simulink model "LTRTenzo"  (R2015a)
settings: Solver=ode23  StartTime=0.0  StopTime=10  RelTol=1e-3
values from neighbouring files (symbols this model uses):
  A0 = tenzo_min_nominale.a    [HTenzoV10.m]    (also in HTenzoV11.m; HTenzoV12.m; HTenzoV13.m; HTenzoV14.m)
  amplitudeNoise = 2    [HTenzoV10.m]    (also in HTenzoV11.m; HTenzoV12.m; HTenzoV13.m; HTenzoV14.m)
  amplitudePertIN = 0    [HTenzoV10.m]    (also in HTenzoV11.m; HTenzoV12.m; HTenzoV13.m; HTenzoV14.m)
  amplitudePertOut = 0    [HTenzoV10.m]    (also in HTenzoV11.m; HTenzoV12.m; HTenzoV13.m; HTenzoV14.m)
  B0 = tenzo_min_nominale.b    [HTenzoV10.m]    (also in HTenzoV11.m; HTenzoV12.m; HTenzoV13.m; HTenzoV14.m)
  C0 = tenzo_min_nominale.c    [HTenzoV10.m]    (also in HTenzoV11.m; HTenzoV12.m; HTenzoV13.m; HTenzoV14.m)
  cstPertIn = 0    [HTenzoV10.m]    (also in HTenzoV11.m; HTenzoV12.m; HTenzoV13.m; HTenzoV14.m)
  cstPertOut = 0    [HTenzoV10.m]    (also in HTenzoV11.m; HTenzoV12.m; HTenzoV13.m; HTenzoV14.m)
  D0 = tenzo_min_nominale.d    [HTenzoV10.m]    (also in HTenzoV11.m; HTenzoV12.m; HTenzoV13.m; HTenzoV14.m)
  KAoss = tenzo_min_nominale.a-L_3*tenzo_min_nominale.c    [HTenzoV12.m]    (also in HTenzoV13.m; HTenzoV14.m; HTenzoV20.m; HTenzoV21.m)
  KBossw = [tenzo_min_nominale.b-L_3*D L_3]    [HTenzoV12.m]    (also in HTenzoV13.m; HTenzoV14.m; HTenzoV20.m; HTenzoV21.m)
  KCoss = eye(size(Aoss,1))    [HTenzoV12.m]    (also in HTenzoV13.m; HTenzoV14.m; HTenzoV20.m; HTenzoV21.m)
  KDoss = zeros(size(Aoss,1),poss)    [HTenzoV12.m]    (also in HTenzoV13.m; HTenzoV14.m; HTenzoV20.m; HTenzoV21.m)
  Kopt = Kopt_3    [HTenzoV10.m]    (also in HTenzoV11.m; HTenzoV12.m; HTenzoV13.m; HTenzoV14.m)
  omegaNoise = 370    [HTenzoV10.m]    (also in HTenzoV11.m; HTenzoV12.m; HTenzoV13.m; HTenzoV14.m)
  omegaPertIN = 6    [HTenzoV10.m]    (also in HTenzoV11.m; HTenzoV12.m; HTenzoV13.m; HTenzoV14.m)
  omegaPertOut = 0.1    [HTenzoV10.m]    (also in HTenzoV11.m; HTenzoV12.m; HTenzoV13.m; HTenzoV14.m)
  randomAmpNoise = 1    [HTenzoV10.m]    (also in HTenzoV11.m; HTenzoV12.m; HTenzoV13.m; HTenzoV14.m)
undefined symbols (not defined in the file or in its folder): sigbuilder_block
settings Model: SimulationMode=accelerator  Creator=danilo  LastModifiedBy=userk
settings OptimizationCC: ExpressionDepthLimit=2147483647
settings DebuggingCC: UnderspecifiedInitializationDetection=Classic  MergeDetectMultiDrivingBlocksExec=none  SolverPrmCheckMsg=warning  FcnCallInpInsideContextMsg=UseLocalSettings  StateNameClashWarn=warning
settings GRTTargetCC: CombineOutputUpdateFcns=off  GRTInterface=on

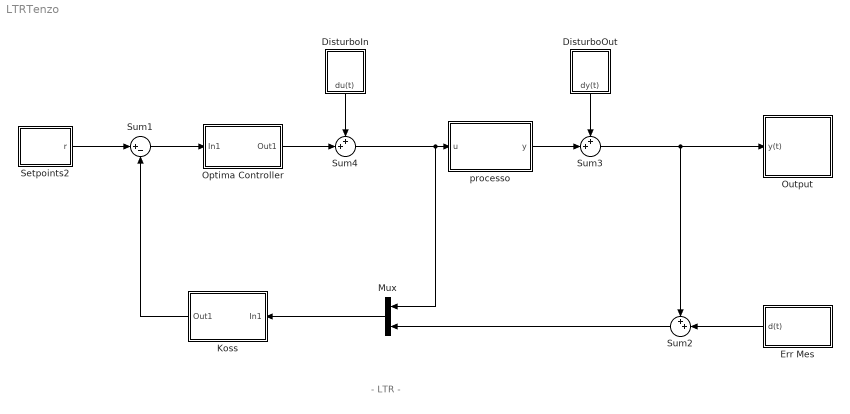
== system LTRTenzo ==
  note: - LTR -
  DisturboIn : Subsystem
  DisturboOut : Subsystem
  Err Mes : Subsystem
  Koss : Subsystem
  Mux : Mux  Inputs=2
  Optima Controller : Subsystem
  Output : Subsystem
  Setpoints2 : Subsystem
  Sum1 : Sum  Inputs=|+-
  Sum2 : Sum  Inputs=++|
  Sum3 : Sum  Inputs=++|
  Sum4 : Sum  Inputs=++|
  processo : Subsystem
  wires:
  Setpoints2/1(r) -> Sum1/1
  Err Mes/1("  d(t)") -> Sum2/2
  Sum2/1 -> Mux/2
  processo/1(y) -> Sum3/2
  DisturboIn/1(du(t)) -> Sum4/1
  Sum3/1 -> Sum2/1, Output/1(y(t))
  DisturboOut/1("dy(t) ") -> Sum3/1
  Sum4/1 -> Mux/1, processo/1(u)
  Sum1/1 -> Optima Controller/1(In1)
  Optima Controller/1(Out1) -> Sum4/2
  Mux/1 -> Koss/1(In1)
  Koss/1(Out1) -> Sum1/2

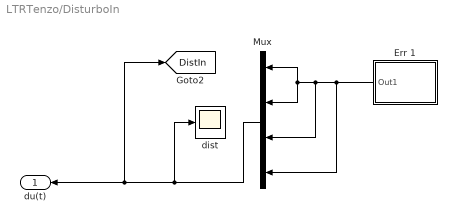
== system LTRTenzo/DisturboIn ==
  Err 1 : Subsystem
  Mux : Mux  Inputs=[1 1 1 1]
  dist : Scope
      settings: SaveName=ScopeData5
  du(t) : Outport
  tag scope: DistIn=global
  wires:
  Mux/1 -> dist/1, [DistIn], du(t)/1
  Err 1/1(Out1) -> Mux/4, Mux/3, Mux/2, Mux/1

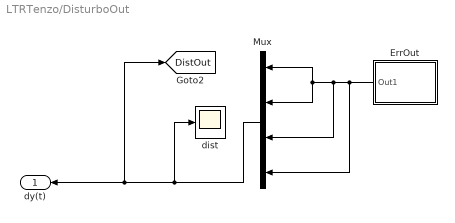
== system LTRTenzo/DisturboOut ==
  ErrOut : Subsystem
  Mux : Mux  Inputs=[1 1 1 1]
  dist : Scope
      settings: TimeRange=50  YMin=-10  YMax=10  SaveName=ScopeData5
  "dy(t) " : Outport
  tag scope: DistOut=global
  wires:
  ErrOut/1(Out1) -> Mux/4, Mux/3, Mux/2, Mux/1
  Mux/1 -> "dy(t) "/1, [DistOut], dist/1

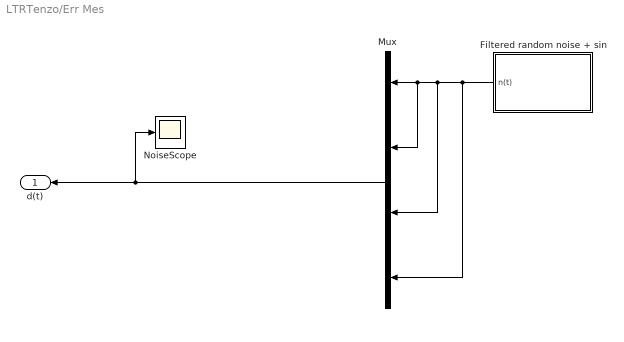
== system LTRTenzo/Err Mes ==
  Filtered random noise + sin : Subsystem
  Mux : Mux  Inputs=[1 1 1 1]
  NoiseScope : Scope
      settings: YMin=-0.004  YMax=0.004  SaveName=ScopeData21
  "  d(t)" : Outport
  wires:
  Mux/1 -> NoiseScope/1, "  d(t)"/1
  Filtered random noise + sin/1(n(t)) -> Mux/4, Mux/3, Mux/2, Mux/1

== system LTRTenzo/Koss ==
  In1 : Inport
  "abc " : StateSpace  A=KAoss  B=KBossw  C=KCoss  D=KDoss  X0=0
  Out1 : Outport
  wires:
  In1/1 -> "abc "/1
  "abc "/1 -> Out1/1

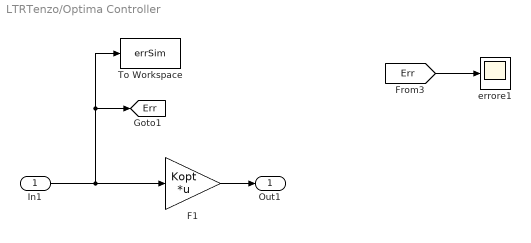
== system LTRTenzo/Optima Controller ==
  In1 : Inport
  F1 : Gain  Gain=Kopt  Multiplication=Matrix(K*u) (u vector)
  To Workspace : ToWorkspace  VariableName=errSim  SaveFormat=Structure  SampleTime=-1
  errore1 : Scope
      settings: ShowLegends=on  YMin=-85  YMax=10  SaveName=ScopeData8
  Out1 : Outport
  tag scope: Err=global
  wires:
  In1/1 -> F1/1, To Workspace/1, [Err]
  F1/1 -> Out1/1
  [Err] -> errore1/1

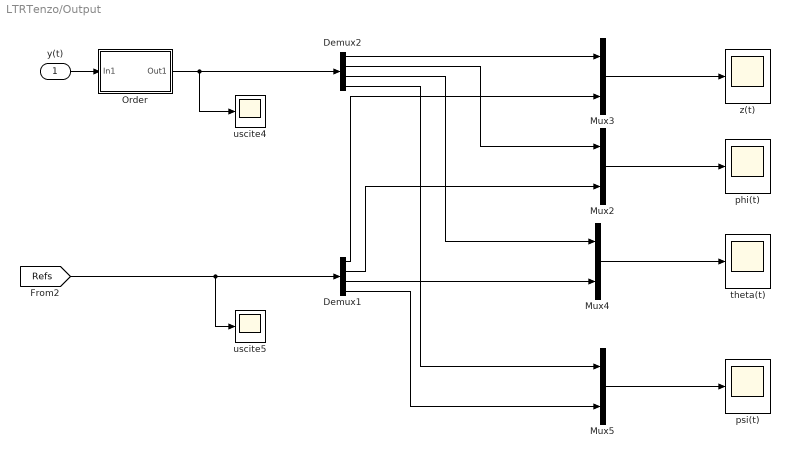
== system LTRTenzo/Output ==
  y(t) : Inport
  Demux1 : Demux
  Demux2 : Demux
  Mux{2..5} (4 alike) : Mux  Inputs=2
  "Order " : Subsystem
  phi(t) : Scope
      settings: TickLabels=on  ShowLegends=on  TimeRange=20  YMin=0  YMax=1700  SaveName=ScopeData4
  psi(t) : Scope
      settings: TickLabels=on  ShowLegends=on  YMin=0.75  YMax=4.25  SaveName=ScopeData7
  theta(t) : Scope
      settings: TickLabels=on  YMin=0  YMax=1700  SaveName=ScopeData6
  uscite4 : Scope
      settings: ShowLegends=on  YMin=675  YMax=975  SaveName=ScopeData2
  uscite5 : Scope
      settings: ShowLegends=on  YMin=675  YMax=975  SaveName=ScopeData9
  z(t) : Scope
      settings: TickLabels=on  ShowLegends=on  YMin=0  YMax=1750
  wires:
  [Refs] -> Demux1/1, uscite5/1
  Demux1/1 -> Mux3/2
  Mux2/1 -> phi(t)/1
  Demux2/2 -> Mux2/1
  Mux3/1 -> z(t)/1
  Demux2/1 -> Mux3/1
  Mux4/1 -> theta(t)/1
  Demux2/3 -> Mux4/1
  Mux5/1 -> psi(t)/1
  Demux2/4 -> Mux5/1
  Demux1/2 -> Mux2/2
  Demux1/3 -> Mux4/2
  Demux1/4 -> Mux5/2
  "Order "/1(Out1) -> Demux2/1, uscite4/1
  y(t)/1 -> "Order "/1(In1)

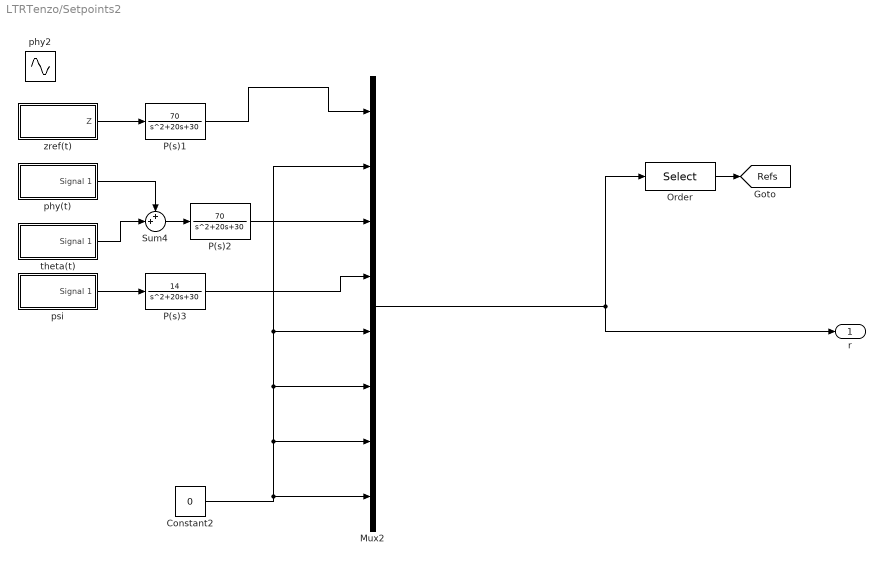
== system LTRTenzo/Setpoints2 ==
  Constant2 : Constant  Value=0
  Mux2 : Mux  Inputs=[1 1 1 1 1 1 1 1]
  Order : Selector  InputPortWidth=8  Indices=[1,3,4,5]
  P(s)1 : TransferFcn  Numerator=70  Denominator=[1 20 30]
  P(s)2 : TransferFcn  Numerator=70  Denominator=[1 20 30]
  P(s)3 : TransferFcn  Numerator=14  Denominator=[1 20 30]
  Sum4 : Sum  Inputs=++|
  phy(t) : Subsystem  Tag=STV Subsys  LoadFcn=sigbuilder_block('load');  StartFcn=sigbuilder_block('start');  StopFcn=sigbuilder_block('stop');  ClipboardFcn=sigbuilder_block('clipboard');  mask(Sigbuilder block){}
      mask help: Simulink:masks:SigbuilderBlock_MD
      mask init:
      | if ~strcmp(get_param(bdroot(gcbh),'SimulationStatus'),'stopped') tuvar = sigbuilder_block('maskInit'); end
      settings: CopyFcn=sigbuilder_block('copy');  DeleteFcn=sigbuilder_block('delete');  ModelCloseFcn=sigbuilder_block('modelClose');  PreSaveFcn=sigbuilder_block('preSave');  PauseFcn=sigbuilder_block('pause');  ContinueFcn=sigbuilder_block('continue');  NameChangeFcn=sigbuilder_block('namechange');  OpenFcn=sigbuilder_block('open',[341.6 120.8 550.4 400 ]);  CloseFcn=sigbuilder_block('close');
      mask Display: plot(0, 0, 100, 100,[2, 2, 32, 32, 2], [68, 8, 8, 68, 68],[32, 2], [38, 38], [32, 19, 2],[53, 60, 44], [32, 17, 17, 2],[16, 16, 31, 31]);txt = getActiveGroup(gcbh);text(2, 100, txt,'verticalAlignment', 'top');
  phy2 : Sin  Amplitude=10  Frequency=0.2  SampleTime=0
  "psi " : Subsystem  Tag=STV Subsys  LoadFcn=sigbuilder_block('load');  StartFcn=sigbuilder_block('start');  StopFcn=sigbuilder_block('stop');  ClipboardFcn=sigbuilder_block('clipboard');  mask(Sigbuilder block){}
      mask help: Simulink:masks:SigbuilderBlock_MD
      mask init:
      | if ~strcmp(get_param(bdroot(gcbh),'SimulationStatus'),'stopped') tuvar = sigbuilder_block('maskInit'); end
      settings: CopyFcn=sigbuilder_block('copy');  DeleteFcn=sigbuilder_block('delete');  ModelCloseFcn=sigbuilder_block('modelClose');  PreSaveFcn=sigbuilder_block('preSave');  PauseFcn=sigbuilder_block('pause');  ContinueFcn=sigbuilder_block('continue');  NameChangeFcn=sigbuilder_block('namechange');  OpenFcn=sigbuilder_block('open',[341.6 120.8 550.4 400 ]);  CloseFcn=sigbuilder_block('close');
      mask Display: plot(0, 0, 100, 100,[2, 2, 32, 32, 2], [68, 8, 8, 68, 68],[32, 2], [38, 38], [32, 19, 2],[53, 60, 44], [32, 17, 17, 2],[16, 16, 31, 31]);txt = getActiveGroup(gcbh);text(2, 100, txt,'verticalAlignment', 'top');
  theta(t) : Subsystem  Tag=STV Subsys  LoadFcn=sigbuilder_block('load');  StartFcn=sigbuilder_block('start');  StopFcn=sigbuilder_block('stop');  ClipboardFcn=sigbuilder_block('clipboard');  mask(Sigbuilder block){}
      mask help: Simulink:masks:SigbuilderBlock_MD
      mask init:
      | if ~strcmp(get_param(bdroot(gcbh),'SimulationStatus'),'stopped') tuvar = sigbuilder_block('maskInit'); end
      settings: CopyFcn=sigbuilder_block('copy');  DeleteFcn=sigbuilder_block('delete');  ModelCloseFcn=sigbuilder_block('modelClose');  PreSaveFcn=sigbuilder_block('preSave');  PauseFcn=sigbuilder_block('pause');  ContinueFcn=sigbuilder_block('continue');  NameChangeFcn=sigbuilder_block('namechange');  OpenFcn=sigbuilder_block('open',[341.6 120.8 550.4 400 ]);  CloseFcn=sigbuilder_block('close');
      mask Display: plot(0, 0, 100, 100,[2, 2, 32, 32, 2], [68, 8, 8, 68, 68],[32, 2], [38, 38], [32, 19, 2],[53, 60, 44], [32, 17, 17, 2],[16, 16, 31, 31]);txt = getActiveGroup(gcbh);text(2, 100, txt,'verticalAlignment', 'top');
  zref(t) : Subsystem  Tag=STV Subsys  LoadFcn=sigbuilder_block('load');  StartFcn=sigbuilder_block('start');  StopFcn=sigbuilder_block('stop');  ClipboardFcn=sigbuilder_block('clipboard');  mask(Sigbuilder block){}
      mask help: Simulink:masks:SigbuilderBlock_MD
      mask init:
      | if ~strcmp(get_param(bdroot(gcbh),'SimulationStatus'),'stopped') tuvar = sigbuilder_block('maskInit'); end
      settings: CopyFcn=sigbuilder_block('copy');  DeleteFcn=sigbuilder_block('delete');  ModelCloseFcn=sigbuilder_block('modelClose');  PreSaveFcn=sigbuilder_block('preSave');  PauseFcn=sigbuilder_block('pause');  ContinueFcn=sigbuilder_block('continue');  NameChangeFcn=sigbuilder_block('namechange');  OpenFcn=sigbuilder_block('open',[341.6 120.8 550.4 400 ]);  CloseFcn=sigbuilder_block('close');
      mask Display: plot(0, 0, 100, 100,[2, 2, 32, 32, 2], [68, 8, 8, 68, 68],[32, 2], [38, 38], [32, 19, 2],[53, 60, 44], [32, 17, 17, 2],[16, 16, 31, 31]);txt = getActiveGroup(gcbh);text(2, 100, txt,'verticalAlignment', 'top');
  r : Outport
  tag scope: Refs=global
  wires:
  theta(t)/1(Signal 1) -> Sum4/2
  phy(t)/1(Signal 1) -> Sum4/1
  Sum4/1 -> P(s)2/1
  P(s)3/1 -> Mux2/4
  P(s)2/1 -> Mux2/3
  P(s)1/1 -> Mux2/1
  "psi "/1(Signal 1) -> P(s)3/1
  Constant2/1 -> Mux2/8, Mux2/7, Mux2/6, Mux2/2, Mux2/5
  zref(t)/1(Z) -> P(s)1/1
  Mux2/1 -> r/1, Order/1
  Order/1 -> [Refs]

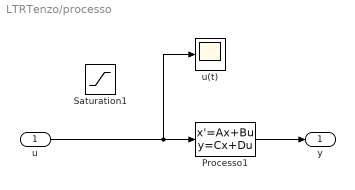
== system LTRTenzo/processo ==
  u : Inport
  Processo1 : StateSpace  A=A0  B=B0  C=C0  D=D0  X0=0
  Saturation1 : Saturate  UpperLimit=7000  LowerLimit=-7000
  "u(t) " : Scope
      settings: SaveName=ScopeData10
  y : Outport
  wires:
  u/1 -> "u(t) "/1, Processo1/1
  Processo1/1 -> y/1

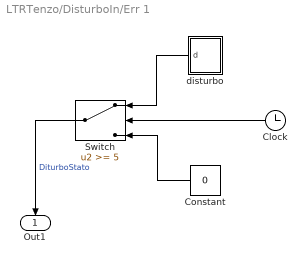
== system LTRTenzo/DisturboIn/Err 1 ==
  Clock : Clock
  Constant : Constant  Value=0
  Switch : Switch  Threshold=5
  disturbo : Subsystem
  Out1 : Outport
  wires:
  Constant/1 -> Switch/3
  disturbo/1(d) -> Switch/1
  Switch/1 -> Out1/1  "DiturboStato"
  Clock/1 -> Switch/2

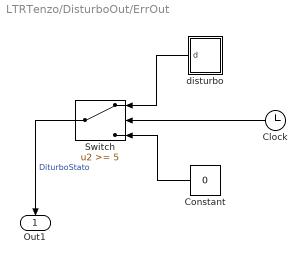
== system LTRTenzo/DisturboOut/ErrOut ==
  Clock : Clock
  Constant : Constant  Value=0
  Switch : Switch  Threshold=5
  disturbo : Subsystem
  Out1 : Outport
  wires:
  Clock/1 -> Switch/2
  Switch/1 -> Out1/1  "DiturboStato"
  disturbo/1(d) -> Switch/1
  Constant/1 -> Switch/3

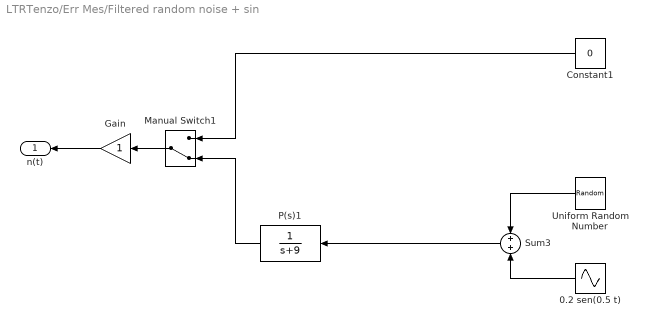
== system LTRTenzo/Err Mes/Filtered random noise + sin ==
  0.2 sen(0.5 t) : Sin  Amplitude=amplitudeNoise  Frequency=omegaNoise  Phase=1  SampleTime=0
  Constant1 : Constant  Value=0
  Gain : Gain
  Manual Switch1 : ManualSwitch  CurrentSetting=0
  P(s)1 : TransferFcn  Numerator=1  Denominator=[1 9]
  Sum3 : Sum
  Uniform Random Number : UniformRandomNumber  Minimum=-randomAmpNoise  Maximum=randomAmpNoise  SampleTime=0.1
  n(t) : Outport
  wires:
  Uniform Random Number/1 -> Sum3/1
  Constant1/1 -> Manual Switch1/1
  Sum3/1 -> P(s)1/1
  Gain/1 -> n(t)/1
  P(s)1/1 -> Manual Switch1/2
  Manual Switch1/1 -> Gain/1
  0.2 sen(0.5 t)/1 -> Sum3/2

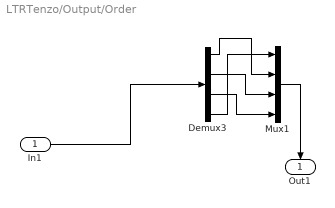
== system LTRTenzo/Output/Order  ==
  In1 : Inport
  Demux3 : Demux
  Mux1 : Mux
  Out1 : Outport
  wires:
  Demux3/2 -> Mux1/3
  Demux3/1 -> Mux1/2
  In1/1 -> Demux3/1
  Mux1/1 -> Out1/1
  Demux3/4 -> Mux1/1
  Demux3/3 -> Mux1/4

== system LTRTenzo/Setpoints2/phy(t) ==
  Demux : Demux  Tag=STV Demux  Outputs=1
  FromWs : FromWorkspace  Tag=STV FromWs  VariableName=tuvar  SampleTime=0
      SigBuilderData=|
      | common.afterFinalStr = 'Extrapolate'
      | common.sampleTime = 0
      | dataSet.timeRange = [0 10]
      | dataSet.name = 'Group 1'
      | sbobj.Groups.Name = 'Group 1'
      | sbobj.Groups.Signals.Name = 'Signal 1'
      | sbobj.Groups.Signals.XData = [0 0.98 2 2 10]
      | sbobj.Groups.Signals.YData = [0 0 50 0 0]
  Signal 1 : Outport  Tag=STV Outport
  wires:
  Demux/1 -> Signal 1/1
  FromWs/1 -> Demux/1

== system LTRTenzo/Setpoints2/psi  ==
  Demux : Demux  Tag=STV Demux  Outputs=1
  FromWs : FromWorkspace  Tag=STV FromWs  VariableName=tuvar  SampleTime=0
      SigBuilderData=|
      | common.afterFinalStr = 'Extrapolate'
      | common.sampleTime = 0
      | dataSet.timeRange = [0 10]
      | dataSet.name = 'Group 1'
      | sbobj.Groups.Name = 'Group 1'
      | sbobj.Groups.Signals.Name = 'Signal 1'
      | sbobj.Groups.Signals.XData = [0 4.06 6.82 10]
      | sbobj.Groups.Signals.YData = [0 190 0 0]
  Signal 1 : Outport  Tag=STV Outport
  wires:
  Demux/1 -> Signal 1/1
  FromWs/1 -> Demux/1

== system LTRTenzo/Setpoints2/theta(t) ==
  Demux : Demux  Tag=STV Demux  Outputs=1
  FromWs : FromWorkspace  Tag=STV FromWs  VariableName=tuvar  SampleTime=0
      SigBuilderData=|
      | common.afterFinalStr = 'Extrapolate'
      | common.sampleTime = 0
      | dataSet.timeRange = [0 10]
      | dataSet.name = 'Group 1'
      | sbobj.Groups.Name = 'Group 1'
      | sbobj.Groups.Signals.Name = 'Signal 1'
      | sbobj.Groups.Signals.XData = [0 1 2.06 4.06 6.82 6.82 10]
      | sbobj.Groups.Signals.YData = [0 0 10 0 20 0 0]
  Signal 1 : Outport  Tag=STV Outport
  wires:
  Demux/1 -> Signal 1/1
  FromWs/1 -> Demux/1

== system LTRTenzo/Setpoints2/zref(t) ==
  Demux : Demux  Tag=STV Demux  Outputs=1
  FromWs : FromWorkspace  Tag=STV FromWs  VariableName=tuvar  SampleTime=0
      SigBuilderData=|
      | common.afterFinalStr = 'Extrapolate'
      | common.sampleTime = 0
      | dataSet.timeRange = [0 10]
      | dataSet.name = 'Group 1'
      | sbobj.Groups.Name = 'Group 1'
      | sbobj.Groups.Signals.Name = 'Z'
      | sbobj.Groups.Signals.XData = [0 1 2.06 4.06 6.82 10]
      | sbobj.Groups.Signals.YData = [0 0 10 10 0 0]
  Z : Outport  Tag=STV Outport
  wires:
  FromWs/1 -> Demux/1
  Demux/1 -> Z/1

== system LTRTenzo/DisturboIn/Err 1/disturbo ==
  Constant : Constant  Value=cstPertIn
  Sine Wave : Sin  Amplitude=amplitudePertIN  Frequency=omegaPertIN  SampleTime=0
  Sum2 : Sum  Inputs=|++
  d : Outport
  wires:
  Sum2/1 -> d/1
  Constant/1 -> Sum2/1
  Sine Wave/1 -> Sum2/2

== system LTRTenzo/DisturboOut/ErrOut/disturbo ==
  Constant : Constant  Value=cstPertOut
  SinOut : Sin  Amplitude=amplitudePertOut  Frequency=omegaPertOut  SampleTime=0
  Sum2 : Sum  Inputs=|++
  d : Outport
  wires:
  SinOut/1 -> Sum2/2
  Constant/1 -> Sum2/1
  Sum2/1 -> d/1
